simulink model "eg_1_03_R2023a"  (R2023a)
settings: Solver=ode4  StartTime=0.0  StopTime=5  FixedStep=0.001  RelTol=1e-3  EnableMultiTasking=on
values from neighbouring files (symbols this model uses):
  A = [  0      1     0      0 ... (first row only)    [eg_1_03b.m]    (also in eg_1_06.m)
  b = [  0 ... (first row only)    [eg_1_03b.m]
  c = [ 0   0   1   0 ]    [eg_1_03b.m]
  h = [ -k  1 ]*inv(M0)*[ zeros(4,1) ... (first row only)    [eg_1_03b.m]
  k = 2    [eg_1_02b.m]    (also in eg_1_03b.m = - lqr(A,b,Q,R); eg_1_05.m; eg_1_06.m)
settings Model: Creator=kawata  LastModifiedBy=kawata
settings SolverCC: AlgebraicLoopSolver=TrustRegion
settings DataIOCC: LimitDataPoints=on  SaveFormat=Array  SignalLoggingSaveFormat=ModelDataLogs  ReturnWorkspaceOutputs=off  SignalLoggingName=sigsOut
settings OptimizationCC: ExpressionDepthLimit=2147483647  LifeSpan=inf
settings DebuggingCC: SaveWithParameterizedLinksMsg=none  UnderspecifiedInitializationDetection=Classic  MergeDetectMultiDrivingBlocksExec=none  SignalResolutionControl=TryResolveAllWithWarning  MultiTaskDSMMsg=warning  MultiTaskCondExecSysMsg=none  FcnCallInpInsideContextMsg=warning  UnconnectedInputMsg=warning  UnconnectedOutputMsg=warning  UnconnectedLineMsg=warning  StateNameClashWarn=warning  SFUnexpectedBacktrackingDiag=warning  SFNoUnconditionalDefaultTransitionDiag=warning  SFExecutionAtInitializationDiag=none  ArithmeticOperatorsInVariantConditions=warning
settings HardwareCC: ProdBitPerPointer=32  ProdBitPerSizeT=32  ProdBitPerPtrDiffT=32  ProdLargestAtomicFloat=None  ProdIntDivRoundTo=Undefined  ProdEndianess=Unspecified  ProdWordSize=32  ProdHWDeviceType=32-bit Generic  TargetUnknown=on
settings ModelReferenceCC: EnableRefExpFcnMdlSchedulingChecks=on  PropagateSignalLabelsOutOfModel=off
settings SFSimCC: SimUseLocalCustomCode=off  CustomCodeUndefinedFunction=UseInterfaceOnly
settings RTWCC: RTWUseLocalCustomCode=off
settings CodeAppCC: StateflowObjectComments=on
settings GRTTargetCC: TargetLangStandard=C89/C90 (ANSI)  CombineOutputUpdateFcns=off  GRTInterface=on
settings ConfigComp: CovMetricSettings=dw  CovSaveCumulativeToWorkspaceVar=on  CovSaveSingleToWorkspaceVar=on  CovExternalEMLEnable=off

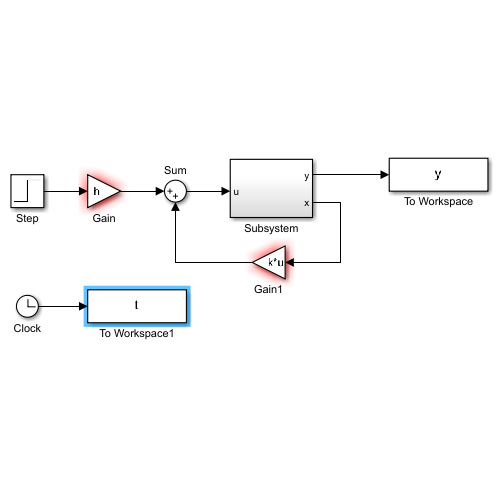
[thumbnail: Simulink's stored preview of the top-level diagram]
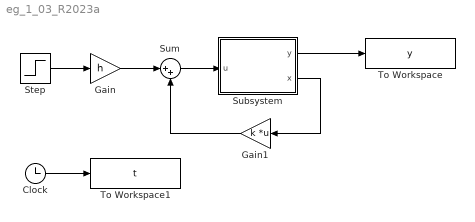
== system eg_1_03_R2023a ==
  Clock : Clock
  Gain : Gain  Gain=h
  Gain1 : Gain  Gain=k  Multiplication=Matrix(K*u)
  Step : Step  Time=0  SampleTime=0
  Subsystem : Subsystem
  Sum : Sum  Inputs=|++  InputSameDT=on  SaturateOnIntegerOverflow=on  OutDataTypeStr=Inherit: Same as first input
  To Workspace : ToWorkspace  VariableName=y  SampleTime=-1
  To Workspace1 : ToWorkspace  VariableName=t  SampleTime=-1
  wires:
  Subsystem/1(y) -> To Workspace/1
  Subsystem/2(x) -> Gain1/1
  Step/1 -> Gain/1
  Gain/1 -> Sum/1
  Sum/1 -> Subsystem/1(u)
  Gain1/1 -> Sum/2
  Clock/1 -> To Workspace1/1

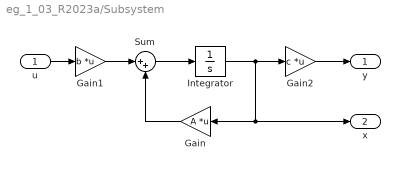
== system eg_1_03_R2023a/Subsystem ==
  u : Inport
  Gain : Gain  Gain=A  Multiplication=Matrix(K*u)
  Gain1 : Gain  Gain=b  Multiplication=Matrix(K*u)
  Gain2 : Gain  Gain=c  Multiplication=Matrix(K*u)
  Integrator : Integrator
  Sum : Sum  Inputs=|++  InputSameDT=on  SaturateOnIntegerOverflow=on  OutDataTypeStr=Inherit: Same as first input
  y : Outport  VectorParamsAs1DForOutWhenUnconnected=off
  x : Outport  Port=2  VectorParamsAs1DForOutWhenUnconnected=off
  wires:
  Gain/1 -> Sum/2
  Sum/1 -> Integrator/1
  Gain1/1 -> Sum/1
  Integrator/1 -> Gain2/1, Gain/1, x/1
  u/1 -> Gain1/1
  Gain2/1 -> y/1
